simulink model "IKS02A1_Mic"  (R2024b)
settings: Solver=FixedStepAuto  StartTime=0.0  StopTime=inf  RelTol=1e-3  EnableMultiTasking=on
PreLoadFcn:
  | addpath(genpath(pwd))
InitFcn:
  | addpath(genpath(pwd));
  | auto_program("IKS02A1_Mic")
  | STLINK_COMPORT = auto_COMPORT()
libraries: instrumentseriallib x3, dspsnks4 x1, dspvision x1
settings Model: SimulationMode=accelerator  ExtModeTrigDuration=10  Creator=JesseJabezArendse  LastModifiedBy=JesseJabezArendse
settings OptimizationCC: ReuseModelBlockBuffer=off  PassReuseOutputArgsAs=Individual arguments  ZeroExternalMemoryAtStartup=off  ZeroInternalMemoryAtStartup=off  MaxStackSize=64  OptimizationLevel=level1  OptimizationCustomize=off  EfficientTunableParamExpr=on
settings DebuggingCC: ParameterPrecisionLossMsg=none  ParameterTunabilityLossMsg=error
settings HardwareCC: ProdBitPerPointer=32  ProdBitPerSizeT=32  ProdBitPerPtrDiffT=32  ProdLargestAtomicInteger=Long  ProdLargestAtomicFloat=Double  ProdWordSize=32  ProdLongLongMode=on  ProdHWDeviceType=ARM Compatible->ARM Cortex
settings ModelReferenceCC: EnableParallelModelReferenceBuilds=on
settings SFSimCC: SimParseCustomCode=off  MATLABDynamicMemAlloc=off  SimHardwareAcceleration=native
settings RTWCC: Description=Embedded Coder  SystemTargetFile=ert.tlc  TemplateMakefile=ert_default_tmf  RTWUseSimCustomCode=on  Toolchain=GNU Tools for ARM Embedded Processors  BuildConfiguration=Specify  GPUComputeCapability=3.5
settings CodeAppCC: ForceParamTrailComments=on  IgnoreCustomStorageClasses=off  OperatorAnnotations=on  SimulinkDataObjDesc=on  SFDataObjDesc=on  InsertBlockDesc=on
settings ERTTargetCC: CodeReplacementLibrary=ARM Cortex-M  SupportContinuousTime=on  ExtModeTransport=3  ExtModeStaticAlloc=on  ExtModeStaticAllocSize=2000  ExtModeMexFile=ext_xcp  ExtModeIntrfLevel=Level2 - Open  InlinedParameterPlacement=Hierarchical  ERTCustomFileTemplate=example_file_process.tlc  DynamicArrayContainerType=coder::array

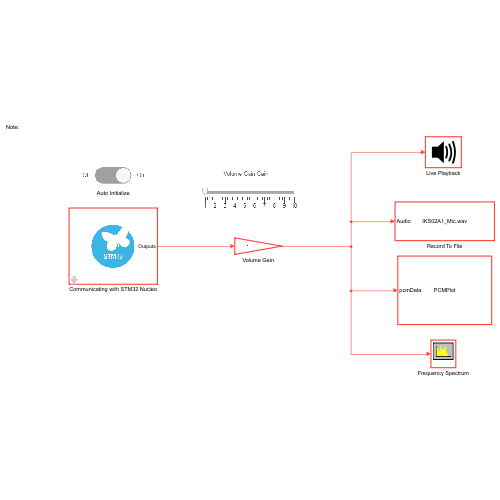
[thumbnail: Simulink's stored preview of the top-level diagram]
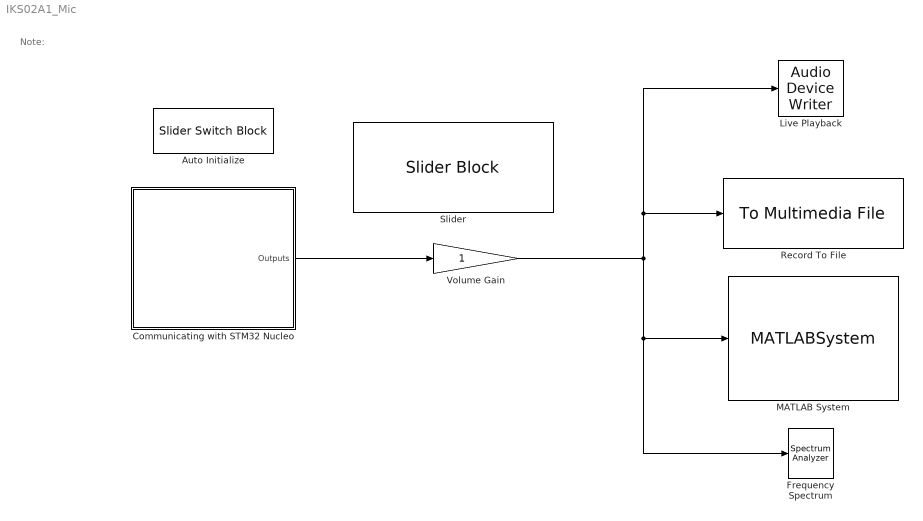
== system IKS02A1_Mic ==
  note: Note:
  Auto Initialize : SliderSwitchBlock  LabelPosition=Hide
      settings: Values={{'Off', 'On'}, [0 1]}
  Communicating with STM32 Nucleo : Subsystem  mask{Auto_Initalize=1}
      mask prompts: Auto_Initalize "Automate Initialization?"
      mask TypeOptions Auto_Initalize: 1 | 0
      mask DialogControl Control1 Prompt: Block for communication between host machine and STM32 Nucleo F411RE
      mask Display: image('stm32_mask_icon.png', [0,0,0,0,80,80]);
  Frequency Spectrum : SpectrumAnalyzer  WindowPosition=[0.000000,36.000000,1536.000000,792.000000,]  Visible=on  ScopeFrameLocation=window  WindowInvariantSamplesPerUpdate=on  Span=81920  StartFrequency=-40960  StopFrequency=40960  YLimits=[-97.72259497,-19.6781853]  SelectedToolstripTab=spectrumAnalyzerToolstrip.measurementsTab
  Live Playback : dspsnks4/Audio Device Writer  Driver=DirectSound  Device=Default  InheritSampleRate=on  SampleRate=44100  BitDepth=16-bit integer  BufferSize=4096  NumBuffers=10  DefaultOutputChannelMapping=on  OutputChannelMapping=1:2  OutputNumUnderrunSamples=off  DriverIdx=1  DeviceWarnFlag=''
  MATLAB System : MATLABSystem  System=PCMPlot
      mask Type: PCMPlot
      mask Display:
      | disp('PCMPlot');
      | port_label('input',1,'pcmData');
  Record To File : dspvision/To Multimedia File  outputFilename=IKS02A1_Mic.wav  streamSelection=Audio only  videoCompressor=None (uncompressed)  audioCompressor=None (uncompressed)  imagePorts=One multidimensional signal  fileType=WAV  audioDatatype=16-bit integer  fourcc=RGB  audioBitRate=128  audioQuality=75  videoQuality=75  mj2000CompFactor=10
      settings: LibrarySourceBlock=dspsnks4/To Multimedia File
  Slider : SliderBlock  ScaleMin=1  ScaleMax=10
  Volume Gain : Gain
  wires:
  Communicating with STM32 Nucleo/1(Outputs) -> Volume Gain/1
  Volume Gain/1 -> Frequency Spectrum/1, MATLAB System/1, Live Playback/1, Record To File/1

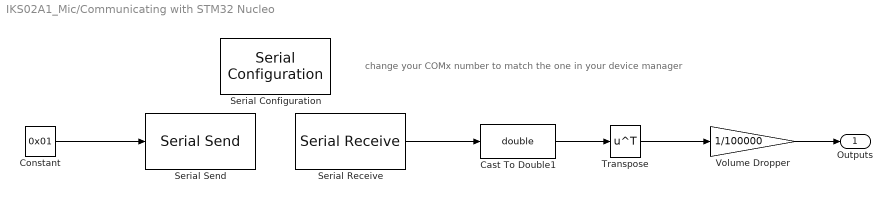
== system IKS02A1_Mic/Communicating with STM32 Nucleo ==
  note: change your COMx number to match the one in your device manager
  Cast To Double1 : DataTypeConversion  OutDataTypeStr=double  SaturateOnIntegerOverflow=off  RndMeth=Floor
  Constant : Constant  Value=0x01
  Serial Configuration : instrumentseriallib/Serial Configuration  Priority=-200000  PortSel=STLINK_COMPORT  Port=STLINK_COMPORT  ComPort=STLINK_COMPORT  BaudRate=921600  DataBits=8  Parity=none  StopBits=1  ByteOrder=big-endian  FlowControl=none  Timeout=5  SimulateUsing=Interpreted execution  BlockInModel=on  aMode=1
      settings: LibrarySourceBlock=embeddedtargetslib/Host Communication/Serial Configuration
  Serial Receive : instrumentseriallib/Serial Receive  Priority=1  PortSel=STLINK_COMPORT  Port=STLINK_COMPORT  ComPort=STLINK_COMPORT  DataType=int16  SaveDataType=uint8  ToggleHeader=off  Header='J_A'  ToggleDataSize=on  DataSize=[1 1600]  ToggleTerminator=off  Terminator=Custom terminator  CustomTerminator='A_J'  InputFormat=Column major  EnableBlockingMode=on  ActionDataUnavailable=Output last received value  ActionWhenDataUnavailable=Output last received value  CustomValue=0  SampleTime=0.1  SimulateUsing=Interpreted execution  BlockInModel=on  aMode=1
      settings: LibrarySourceBlock=embeddedtargetslib/Host Communication/Serial Receive
  Serial Send : instrumentseriallib/Serial Send  Priority=1  PortSel=COM10  Port=COM10  ComPort=COM10  Header=[]  Terminator=<none>  CustomTerminator=[]  EnableBlockingMode=on  SimulateUsing=Interpreted execution  BlockInModel=on  aMode=1
      settings: LibrarySourceBlock=embeddedtargetslib/Host Communication/Serial Send
  Transpose : Math  Operator=transpose
  Volume Dropper : Gain  Gain=1/100000
  Outputs : Outport
  wires:
  Serial Receive/1 -> Cast To Double1/1
  Constant/1 -> Serial Send/1
  Cast To Double1/1 -> Transpose/1
  Transpose/1 -> Volume Dropper/1
  Volume Dropper/1 -> Outputs/1
